simulink model "tilting_NMPC"  (R2023b)
settings: Solver=VariableStepAuto  StartTime=0.0  StopTime=tot_time  RelTol=1e-3
PreLoadFcn:
  | mainNMPC
InitFcn:
  | addpath('TRAJECTORIES\');
  | square_tilting
  | %circular_coplanar
StartFcn:
  | %% Setup Video e Timer
  | videoFile = 'NMPC_quad.avi';
  | %videoFile = 'NMPC_circ.avi';
  | videoObj = VideoWriter(videoFile);
  | videoObj.FrameRate = 30;
  | open(videoObj);
  | assignin('base','videoObj',videoObj);
  | 
  | 
  | t = timer('ExecutionMode','fixedSpacing','Period',0.05,'StartDelay',2,...
  |           'TimerFcn',@(~,~) captureFrame(findall(0,'Type','figure','Name','UAV Animation'), videoObj));
  | start(t);
  | 
  | 
  | assignin('base','videoTimer',t);
StopFcn:
  | % Default graphics settings
  | set(0, 'DefaultTextInterpreter', 'latex')
  | set(0, 'DefaultLegendInterpreter', 'latex')
  | set(0, 'DefaultAxesTickLabelInterpreter', 'latex')
  | lw = 2;
  | plot_errors = figure('Renderer', 'painters', 'Position', [10 10 900 650]);
  | subplot(2,1,1)
  | plot(out.err_p.time, out.err_p.signals.values(1,:), 'k-', 'Linewidth', lw ,'Color', [0.2, 0.2, 0.2]);
  | hold on
  | plot(out.err_p.time, out.err_p.signals.values(2,:), 'k-', 'Linewidth', lw ,'Color', [1, 0, 0]);
  | hold on
  | plot(out.err_p.time, out.err_p.signals.values(3,:), 'k-', 'Linewidth', lw ,'Color', [0, 0, 1]);
  | legend({'x-axis', 'y-axis', 'z-axis'}, ...
  |        'Location', 'southwest', ...
  |        'Orientation', 'vertical', ...
  |        'FontSize', 9);
  | %xlabel('Time [s]')
  | ylabel('$e_p$ [m]')
  | set(gca, 'FontSize',18);
  | %Grid
  | grid on
  | box on
  | %----------------------------------------------------------
  | subplot(2,1,2)
  | plot(out.dot_err_p.time, out.dot_err_p.signals.values(1,:), 'k-', 'Linewidth', lw ,'Color', [0.2, 0.2, 0.2]);
  | hold on
  | plot(out.dot_err_p.time, out.dot_err_p.signals.values(2,:), 'k-', 'Linewidth', lw ,'Color', [1, 0, 0]);
  | hold on
  | plot(out.dot_err_p.time, out.dot_err_p.signals.values(3,:), 'k-', 'Linewidth', lw ,'Color', [0, 0, 1]);
  | legend({'x-axis', 'y-axis', 'z-axis'}, ...
  |        'Location', 'northeast', ...
  |        'Orientation', 'vertical', ...
  |        'FontSize', 10);
  | 
  | ylabel('$\dot{e}_p$ [m/s]')
  | xlabel('Time [s]');
  | set(gca, 'FontSize',18);
  | %Grid
  | grid on
  | box on
  | 
  | exportgraphics(plot_errors, 'Tilting_MPC_cer_lin_err.pdf');
  | %--------------------------------------------------
  | plot_errors_or = figure('Renderer', 'painters', 'Position', [10 10 900 650]);
  | subplot(2,1,1)
  | plot(out.eR.time, out.eR.signals.values(1,:), 'k-', 'Linewidth', lw ,'Color', [0.2, 0.2, 0.2]);
  | hold on
  | plot(out.eR.time, out.eR.signals.values(2,:), 'k-', 'Linewidth', lw ,'Color', [1, 0, 0]);
  | hold on
  | plot(out.eR.time, out.eR.signals.values(3,:), 'k-', 'Linewidth', lw ,'Color', [0, 0, 1]);
  | legend({'x-axis', 'y-axis', 'z-axis'}, ...
  |        'Location', 'northeast', ...
  |        'Orientation', 'vertical', ...
  |        'FontSize', 10);
  | ylabel('$e_R$ [rad]')
  | set(gca, 'FontSize',18);
  | %Grid
  | grid on
  | box on
  | %----------------------------------------------------------
  | subplot(2,1,2)
  | plot(out.ew.time, out.ew.signals.values(1,:), 'k-', 'Linewidth', lw ,'Color', [0.2, 0.2, 0.2]);
  | hold on
  | plot(out.ew.time, out.ew.signals.values(2,:), 'k-', 'Linewidth', lw ,'Color', [1, 0, 0]);
  | hold on
  | plot(out.ew.time, out.ew.signals.values(3,:), 'k-', 'Linewidth', lw ,'Color', [0, 0, 1]);
  | legend({'x-axis', 'y-axis', 'z-axis'}, ...
  |        'Location', 'northeast', ...
  |        'Orientation', 'vertical', ...
  |        'FontSize', 10);
  | 
  | ylabel('$e_\omega$ [rad/s]')
  | xlabel('Time [s]');
  | set(gca, 'FontSize',18);
  | %Grid
  | grid on
  | box on
  | 
  | exportgraphics(plot_errors_or, 'Tilting_MPC_cer_or_err.pdf');
  | %---------------------------------------------------------------------
  | plot_v = figure('Renderer', 'painters', 'Position', [10 10 900 300]);
  | plot(out.v.time, out.v.signals.values(:,3), 'k-', 'Linewidth', lw ,'Color', [0.2, 0.2, 0.2]);
  | xlabel('Time [s]')
  | ylabel('$f_z$ [N]')
  | set(gca, 'FontSize',18);
  | %Grid
  | grid on
  | box on
  | %Options
  | set(gcf,'color','w');
  | set(plot_v, 'MenuBar', 'none', 'ToolBar', 'none');
  | exportgraphics(plot_v, 'Tilting_MPC_cer_fz.pdf');
  | 
  | %---------------------
  | 
  | videoObj = evalin('base','videoObj');
  | t = evalin('base','videoTimer');
  | 
  | 
  | stop(t);
  | delete(t);
  | close(videoObj);
  | 
  | 
  | clear videoObj videoTimer
  | disp('Saved Video UAV');
undefined symbols (not defined in the file or in its folder): Ts
libraries: robotcorelib x2, mpclib x1, matrix_library x1, uavutilslib x1
settings Model: SimulationMode=accelerator  Creator=acer  LastModifiedBy=laura

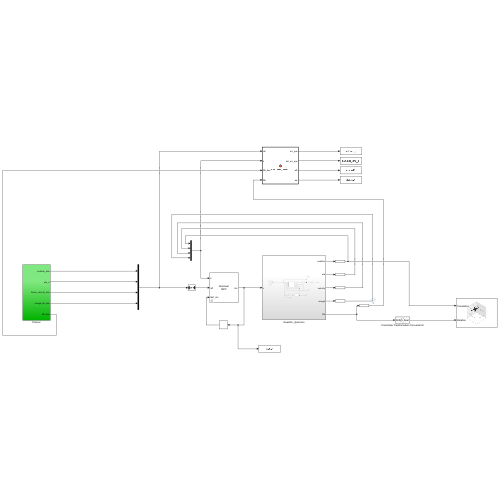
[thumbnail: Simulink's stored preview of the top-level diagram]
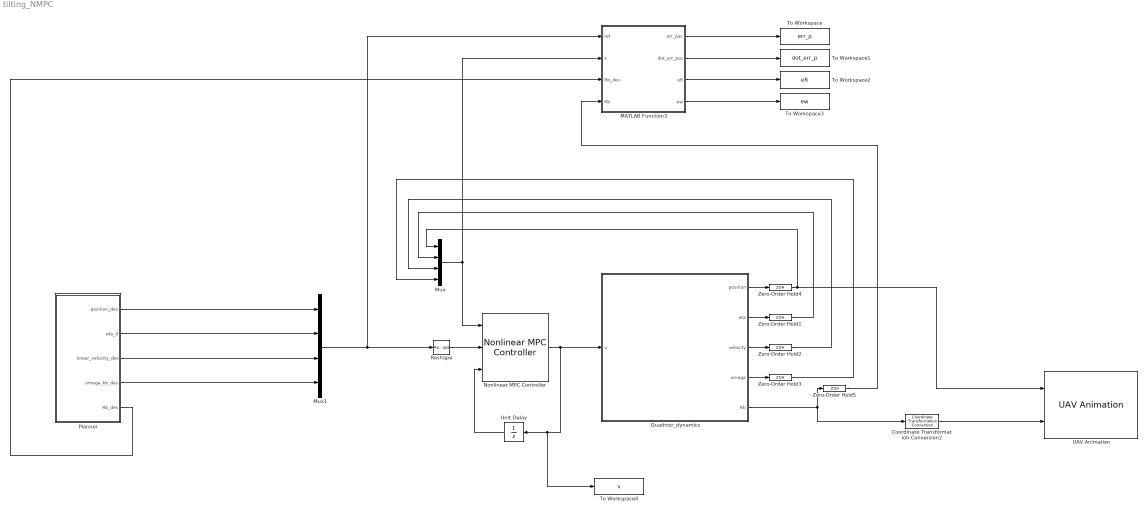
== system tilting_NMPC ==
  Coordinate Transformation Conversion2 : robotcorelib/Coordinate Transformation Conversion  InputRepresentation=Rotation Matrix  InputEulerSequence=ZYX  ShowTrVecInputPort=on  OutputRepresentation=Quaternion  OutputEulerSequence=ZYX  ShowTrVecOutputPort=on  SimulateUsing=Interpreted execution
  MATLAB Function3 : MATLAB Function  TreatAsAtomicUnit=on
  Mux : Mux  Inputs=[3, 3, 3, 3]
  Mux1 : Mux  Inputs=[3, 3, 3, 3]
  Nonlinear MPC Controller : mpclib/Nonlinear MPC Controller  nlmpcobj=nlobjecto  UseObjectTs=on  UseMEX=off  md_enabled=off  mvtarget_enabled=off  param_enabled=off  cost_enabled=off  mvseq_enabled=off  stateseq_enabled=off  ovseq_enabled=off  slack_enabled=off  status_enabled=off  ov_min=off  ov_max=off  mv_min=off  mv_max=off  mvrate_min=off  mvrate_max=off  state_min=off  state_max=off  ov_weight=off  mv_weight=off  mvrate_weight=off  ecr_weight=off  nlp_initialize=off
  Planner : Subsystem
  Quadrtor_dynamics : Subsystem
  Reshape : Reshape  OutputDimensionality=Row vector (2-D)  OutputDimensions=[1,12]
  To Workspace : ToWorkspace  VariableName=err_p  SaveFormat=Structure With Time  SampleTime=-1
  To Workspace1 : ToWorkspace  VariableName=dot_err_p  SaveFormat=Structure With Time  SampleTime=-1
  To Workspace2 : ToWorkspace  VariableName=eR  SaveFormat=Structure With Time  SampleTime=-1
  To Workspace3 : ToWorkspace  VariableName=ew  SaveFormat=Structure With Time  SampleTime=-1
  To Workspace4 : ToWorkspace  VariableName=v  SaveFormat=Structure With Time  SampleTime=-1
  UAV Animation : uavutilslib/UAV Animation  UAVType=Multirotor  UAVSize=1  InertialZDirection=Down  SampleTime=0.01
  Unit Delay : UnitDelay  InitialCondition=[0 0 -13 0 0 0]'  SampleTime=Ts  HasFrameUpgradeWarning=on
  Zero-Order Hold{1..5} (5 alike) : ZeroOrderHold  SampleTime=Ts
  wires:
  Unit Delay/1 -> Nonlinear MPC Controller/3
  Planner/1(position_des) -> Mux1/1
  Planner/2(eta_d) -> Mux1/2
  Planner/3(linear_velocity_des) -> Mux1/3
  Planner/4(omega_bb_des) -> Mux1/4
  Coordinate Transformation Conversion2/1 -> UAV Animation/2
  Mux1/1 -> Reshape/1, MATLAB Function3/1(ref)
  Reshape/1 -> Nonlinear MPC Controller/2
  Nonlinear MPC Controller/1 -> To Workspace4/1, Unit Delay/1, Quadrtor_dynamics/1(v)
  Zero-Order Hold1/1 -> Mux/2
  Planner/5(Rb_des) -> MATLAB Function3/3(Rb_des)
  Zero-Order Hold3/1 -> Mux/4
  Mux/1 -> MATLAB Function3/2(x), Nonlinear MPC Controller/1
  MATLAB Function3/1(err_pos) -> To Workspace/1
  MATLAB Function3/3(eR) -> To Workspace2/1
  MATLAB Function3/4(ew) -> To Workspace3/1
  Quadrtor_dynamics/1(position) -> Zero-Order Hold4/1
  Quadrtor_dynamics/3(velocity) -> Zero-Order Hold2/1
  Quadrtor_dynamics/2(eta) -> Zero-Order Hold1/1
  Zero-Order Hold2/1 -> Mux/3
  Quadrtor_dynamics/4(omega) -> Zero-Order Hold3/1
  Quadrtor_dynamics/5(Rb) -> Coordinate Transformation Conversion2/1, Zero-Order Hold5/1
  Zero-Order Hold5/1 -> MATLAB Function3/4(Rb)
  Zero-Order Hold4/1 -> Mux/1, UAV Animation/1
  MATLAB Function3/2(dot_err_pos) -> To Workspace1/1

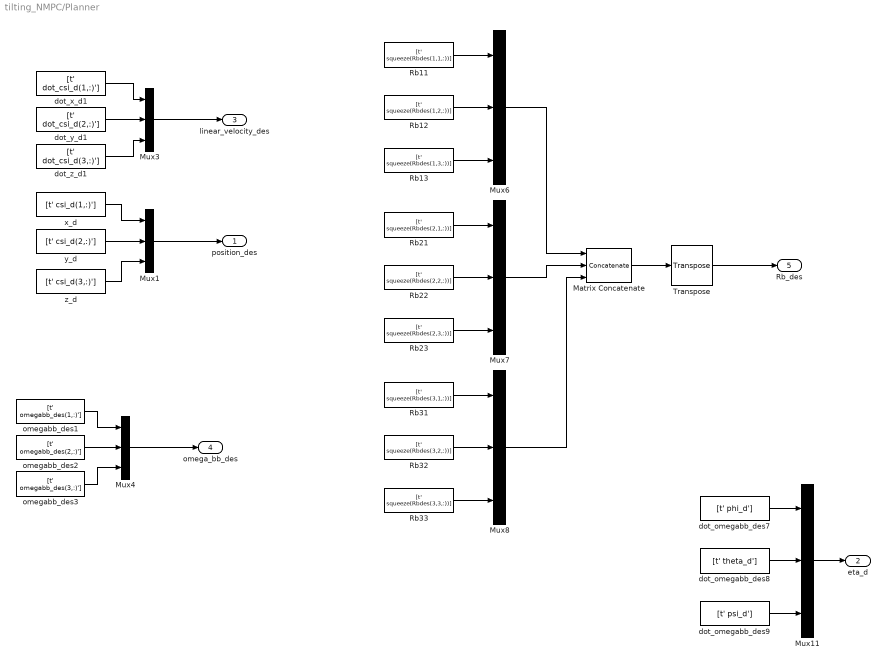
== system tilting_NMPC/Planner ==
  Matrix Concatenate : Concatenate  NumInputs=3  Mode=Multidimensional array  ConcatenateDimension=2
  Mux{1,3..4,6..8,11} (7 alike) : Mux  Inputs=3
  Rb11 : FromWorkspace  VariableName=[t' squeeze(Rbdes(1,1,:))]  SampleTime=Ts
  Rb12 : FromWorkspace  VariableName=[t' squeeze(Rbdes(1,2,:))]  SampleTime=Ts
  Rb13 : FromWorkspace  VariableName=[t' squeeze(Rbdes(1,3,:))]  SampleTime=Ts
  Rb21 : FromWorkspace  VariableName=[t' squeeze(Rbdes(2,1,:))]  SampleTime=Ts
  Rb22 : FromWorkspace  VariableName=[t' squeeze(Rbdes(2,2,:))]  SampleTime=Ts
  Rb23 : FromWorkspace  VariableName=[t' squeeze(Rbdes(2,3,:))]  SampleTime=Ts
  Rb31 : FromWorkspace  VariableName=[t' squeeze(Rbdes(3,1,:))]  SampleTime=Ts
  Rb32 : FromWorkspace  VariableName=[t' squeeze(Rbdes(3,2,:))]  SampleTime=Ts
  Rb33 : FromWorkspace  VariableName=[t' squeeze(Rbdes(3,3,:))]  SampleTime=Ts
  Transpose : matrix_library/Transpose
  dot_omegabb_des7 : FromWorkspace  VariableName=[t' phi_d']  SampleTime=Ts
  dot_omegabb_des8 : FromWorkspace  VariableName=[t' theta_d']  SampleTime=Ts
  dot_omegabb_des9 : FromWorkspace  VariableName=[t' psi_d']  SampleTime=Ts
  dot_x_d1 : FromWorkspace  VariableName=[t' dot_csi_d(1,:)']  SampleTime=Ts
  dot_y_d1 : FromWorkspace  VariableName=[t' dot_csi_d(2,:)']  SampleTime=Ts
  dot_z_d1 : FromWorkspace  VariableName=[t' dot_csi_d(3,:)']  SampleTime=Ts
  omegabb_des1 : FromWorkspace  VariableName=[t' omegabb_des(1,:)']  SampleTime=Ts
  omegabb_des2 : FromWorkspace  VariableName=[t' omegabb_des(2,:)']  SampleTime=Ts
  omegabb_des3 : FromWorkspace  VariableName=[t' omegabb_des(3,:)']  SampleTime=Ts
  x_d : FromWorkspace  VariableName=[t' csi_d(1,:)']  SampleTime=Ts
  y_d : FromWorkspace  VariableName=[t' csi_d(2,:)']  SampleTime=Ts
  z_d : FromWorkspace  VariableName=[t' csi_d(3,:)']  SampleTime=Ts
  position_des : Outport
  eta_d : Outport  Port=2
  linear_velocity_des : Outport  Port=3
  omega_bb_des : Outport  Port=4
  Rb_des : Outport  Port=5
  wires:
  y_d/1 -> Mux1/2
  z_d/1 -> Mux1/3
  x_d/1 -> Mux1/1
  Mux1/1 -> position_des/1
  dot_y_d1/1 -> Mux3/2
  dot_z_d1/1 -> Mux3/3
  dot_x_d1/1 -> Mux3/1
  Mux3/1 -> linear_velocity_des/1
  omegabb_des3/1 -> Mux4/3
  Mux4/1 -> omega_bb_des/1
  omegabb_des2/1 -> Mux4/2
  omegabb_des1/1 -> Mux4/1
  Rb11/1 -> Mux6/1
  Rb12/1 -> Mux6/2
  Rb13/1 -> Mux6/3
  Rb23/1 -> Mux7/3
  Rb22/1 -> Mux7/2
  Rb21/1 -> Mux7/1
  Rb31/1 -> Mux8/1
  Rb32/1 -> Mux8/2
  Rb33/1 -> Mux8/3
  Mux6/1 -> Matrix Concatenate/1
  Mux7/1 -> Matrix Concatenate/2
  Mux8/1 -> Matrix Concatenate/3
  Matrix Concatenate/1 -> Transpose/1
  Transpose/1 -> Rb_des/1
  Mux11/1 -> eta_d/1
  dot_omegabb_des9/1 -> Mux11/3
  dot_omegabb_des8/1 -> Mux11/2
  dot_omegabb_des7/1 -> Mux11/1

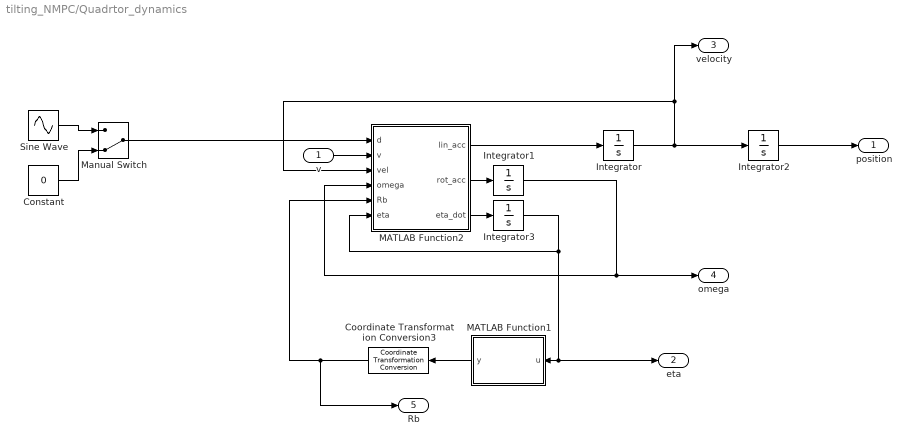
== system tilting_NMPC/Quadrtor_dynamics ==
  v : Inport
  Constant : Constant  Value=0
  Coordinate Transformation Conversion3 : robotcorelib/Coordinate Transformation Conversion  InputRepresentation=Euler Angles  InputEulerSequence=ZYX  ShowTrVecInputPort=on  OutputRepresentation=Rotation Matrix  OutputEulerSequence=ZYX  ShowTrVecOutputPort=on  SimulateUsing=Interpreted execution
  Integrator : Integrator  InitialCondition=[0 0 0]'
  Integrator1 : Integrator  InitialCondition=[0 0 0]'
  Integrator2 : Integrator  InitialCondition=[0 0 -1]'
  Integrator3 : Integrator  InitialCondition=[0 0 0]'
  MATLAB Function1 : MATLAB Function  TreatAsAtomicUnit=on
  MATLAB Function2 : MATLAB Function  TreatAsAtomicUnit=on
  Manual Switch : ManualSwitch  CurrentSetting=0
  Sine Wave : Sin  Frequency=0.2  SampleTime=0
  position : Outport
  eta : Outport  Port=2
  velocity : Outport  Port=3
  omega : Outport  Port=4
  Rb : Outport  Port=5
  wires:
  MATLAB Function2/2(rot_acc) -> Integrator1/1
  Coordinate Transformation Conversion3/1 -> Rb/1, MATLAB Function2/5(Rb)
  MATLAB Function2/1(lin_acc) -> Integrator/1
  Integrator1/1 -> omega/1, MATLAB Function2/4(omega)
  Integrator3/1 -> MATLAB Function1/1(u), eta/1, MATLAB Function2/6(eta)
  Integrator2/1 -> position/1
  MATLAB Function2/3(eta_dot) -> Integrator3/1
  v/1 -> MATLAB Function2/2(v)
  MATLAB Function1/1(y) -> Coordinate Transformation Conversion3/1
  Integrator/1 -> velocity/1, MATLAB Function2/3(vel), Integrator2/1
  Sine Wave/1 -> Manual Switch/1
  Constant/1 -> Manual Switch/2
  Manual Switch/1 -> MATLAB Function2/1(d)

== matlab function tilting_NMPC/MATLAB Function3 ==
  data: ref input; x input; Rb_des input; err_pos output; dot_err_pos output; eR output; ew output; Rb input
function [err_pos,dot_err_pos, eR, ew] = compute_errors(ref,x,Rb_des,Rb)
    pos = x(1:3);
    eta = x(4:6);
    vel = x(7:9);
    omega = x(10:12);

    pos_des = ref(1:3);
    eta_des = ref(4:6);
    vel_des = ref(7:9);
    omega_des = ref(10:12);
    
    %Compute errors
    err_pos = pos - pos_des;
    dot_err_pos = vel - vel_des;

    eR = 0.5*vee(Rb_des'*Rb - Rb'*Rb_des);
    ew = omega - Rb'*Rb_des*omega_des;
   
end

function S = skew(v)
    if(numel(v)~= 1)
    S= [0 -v(3) v(2);
        v(3) 0 -v(1);
        -v(2) v(1) 0];
    else
    S= zeros(3);
    end
end

function v = vee(S)
    v = [S(3,2); S(1,3); S(2,1)];
end

== matlab function tilting_NMPC/Quadrtor_dynamics/MATLAB Function1 ==
  data: u input; y output
function y = fcn(u)

y = [u(3) u(2) u(1)]';

== matlab function tilting_NMPC/Quadrtor_dynamics/MATLAB Function2 ==
  data: d input; v input; lin_acc output; vel input; rot_acc output; omega input; Rb input; eta_dot output; eta input
function [lin_acc, rot_acc, eta_dot] = fcn(d,v, vel,omega, Rb, eta)

g = [0 0 9.81]';
m = 1.32;
AT = diag([0.9 0.9 0.75]);
AR = diag([0.6 0.6 0.6]);
J = diag([0.0154 0.0154 0.0263]);

H = [1 sin(eta(1))*tan(eta(2)) cos(eta(1))*tan(eta(2));
     0 cos(eta(1)) -sin(eta(1));
     0 sin(eta(1))/cos(eta(2)) cos(eta(1))/cos(eta(2))];

eta_dot=H*omega;

prod_vec = [-omega(2)*omega(3)*(J(3,3)-J(2,2));
            -omega(3)*omega(1)*(J(1,1)-J(3,3));
            -omega(1)*omega(2)*(J(2,2)-J(1,1))];

fP = [v(1) v(2) v(3)]';
tauP = [v(4) v(5) v(6)]';

fD=d*ones(3,1);
tauD=zeros(3,1);

lin_acc = g+(1/m)*(Rb*fP-Rb*AT*vel+fD);
rot_acc = inv(J)*(prod_vec+tauP-AR*omega+tauD);

end

function S = skew(v)
if(numel(v)~= 1)
S= [0 -v(3) v(2); 
    v(3) 0 -v(1);
    -v(2) v(1) 0];
else
S= zeros(3);
end
end
